simulink model "Simulink_PLC_coder_example"  (R2024a)
settings: Solver=FixedStepDiscrete  StartTime=0.0  StopTime=10  FixedStep=0.0001  RelTol=1e-3
settings Model: Creator=Jan Størbu  LastModifiedBy=Are-Laptop
settings SolverCC: AlgebraicLoopSolver=TrustRegion
settings DataIOCC: ReturnWorkspaceOutputs=off
settings DebuggingCC: UnconnectedInputMsg=warning  UnconnectedOutputMsg=warning  UnconnectedLineMsg=warning  BusObjectLabelMismatch=error  ArithmeticOperatorsInVariantConditions=warning
settings ModelReferenceCC: EnableRefExpFcnMdlSchedulingChecks=on
settings SFSimCC: SimUseLocalCustomCode=off  CustomCodeUndefinedFunction=UseInterfaceOnly
settings RTWCC: RTWUseLocalCustomCode=off  GPUComputeCapability=3.5  DLArmComputeVersion=19.05
settings ConfigComp: PLC_TargetIDE=plcopen  PLC_MultiTBSigbuilderTimeRange=off  PLC_ReuseMLFcnVariable=on  PLC_FoldFBCallOutputVar=off  PLC_RemoveUnusedSSMethodCallArguments=off  PLC_UseCallOutputArgSyntax=off  PLC_EnableUnsignedAndDoubleTypes=off  PLC_EnableUDTSplitting=off  PLC_MaxFieldsInUDT=500  PLC_InlineEnumCastFunction=off  PLC_GenerateReport=off  PLC_LaunchReport=off

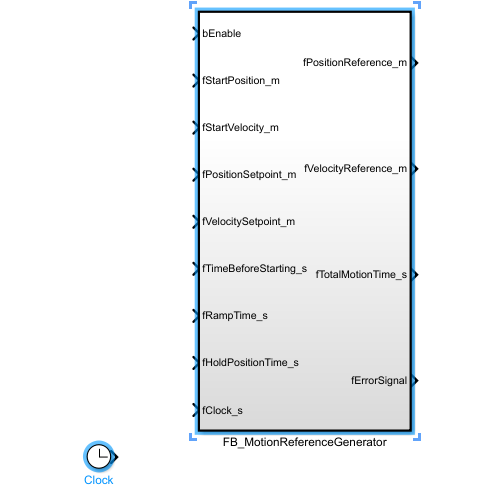
[thumbnail: Simulink's stored preview of the top-level diagram]
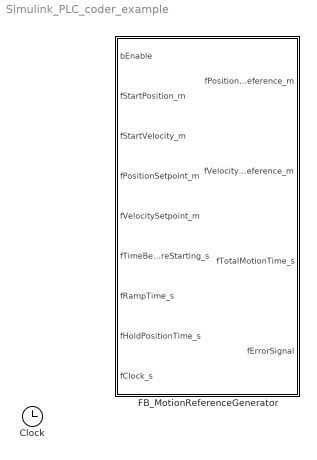
== system Simulink_PLC_coder_example ==
  Clock : Clock
  FB_MotionReferenceGenerator : Subsystem  TreatAsAtomicUnit=on  VariantControl=Ramp_Profile

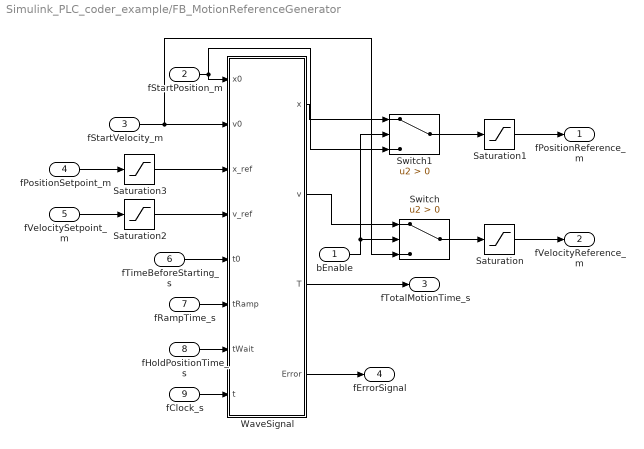
== system Simulink_PLC_coder_example/FB_MotionReferenceGenerator ==
  bEnable : Inport  OutDataTypeStr=boolean
  fStartPosition_m : Inport  Port=2
  fStartVelocity_m : Inport  Port=3
  fPositionSetpoint_m : Inport  Port=4
  fVelocitySetpoint_m : Inport  Port=5
  fTimeBeforeStarting_s : Inport  Port=6
  fRampTime_s : Inport  Port=7
  fHoldPositionTime_s : Inport  Port=8
  fClock_s : Inport  Port=9
  Saturation : Saturate  UpperLimit=0.05  LowerLimit=-0.05
  Saturation1 : Saturate  UpperLimit=0.45  LowerLimit=0
  Saturation2 : Saturate  UpperLimit=0.05  LowerLimit=0
  Saturation3 : Saturate  UpperLimit=0.45  LowerLimit=0
  Switch : Switch  Criteria=u2 > Threshold  SaturateOnIntegerOverflow=off  InputSameDT=off
  Switch1 : Switch  Criteria=u2 > Threshold  SaturateOnIntegerOverflow=off  InputSameDT=off
  WaveSignal : MATLAB Function  TreatAsAtomicUnit=on
  fPositionReference_m : Outport  VectorParamsAs1DForOutWhenUnconnected=off
  fVelocityReference_m : Outport  Port=2  VectorParamsAs1DForOutWhenUnconnected=off
  fTotalMotionTime_s : Outport  Port=3  VectorParamsAs1DForOutWhenUnconnected=off
  fErrorSignal : Outport  Port=4  VectorParamsAs1DForOutWhenUnconnected=off
  wires:
  fClock_s/1 -> WaveSignal/8(t)
  WaveSignal/2(v) -> Switch/1
  Switch/1 -> Saturation/1
  fStartVelocity_m/1 -> Switch/3, WaveSignal/2(v0)
  fTimeBeforeStarting_s/1 -> WaveSignal/5(t0)
  fPositionSetpoint_m/1 -> Saturation3/1
  fHoldPositionTime_s/1 -> WaveSignal/7(tWait)
  fVelocitySetpoint_m/1 -> Saturation2/1
  WaveSignal/1(x) -> Switch1/1
  WaveSignal/3(T) -> fTotalMotionTime_s/1
  fStartPosition_m/1 -> Switch1/3, WaveSignal/1(x0)
  Switch1/1 -> Saturation1/1
  Saturation/1 -> fVelocityReference_m/1
  Saturation2/1 -> WaveSignal/4(v_ref)
  Saturation3/1 -> WaveSignal/3(x_ref)
  fRampTime_s/1 -> WaveSignal/6(tRamp)
  WaveSignal/4(Error) -> fErrorSignal/1
  Saturation1/1 -> fPositionReference_m/1
  bEnable/1 -> Switch1/2, Switch/2

== matlab function Simulink_PLC_coder_example/FB_MotionReferenceGenerator/WaveSignal ==
  data: x0 input; v0 input; x_ref input; x output; v_ref input; t0 input; tRamp input; tWait input; v output; t input; T output; Error output double
function [x,v,T, Error] = fcn(x0,v0, x_ref,v_ref,t0,tRamp,tWait,t)
x_SP = x_ref - x0;
vs=v_ref;
slopeExt=v0-vs;
slopeRetr=-vs-v0;

as = vs/tRamp;
s_acc=(vs^2-v0^2)/as;

tHold=(x_SP-s_acc)/vs;

if tHold < 0 
Error = 1;
else 
Error = 0;
end

t1=tRamp;
t2=tHold; 
t3=tRamp;
t4=tWait;
t5=t1;
t6=t2;
t7=t3;

x = x0;
x1 = x0 + v0*((t0+t1)-t0)-(slopeExt/t1)*((t0+t1)-t0)^2/2;
x2 = x1 + vs*((t0+t1+t2)-(t0+t1)); 
x4 = x_ref - v0*((t0+t1+t2+t3+t4+t5)-(t0+t1+t2+t3+t4))+(slopeRetr/t5)*((t0+t1+t2+t3+t4+t5)-(t0+t1+t2+t3+t4))^2/2; 
x5 = x4-vs*((t0+t1+t2+t3+t4+t5+t6)-(t0+t1+t2+t3+t4+t5));  

if Error == 1
x = x0;
v = v0; 
elseif t>=0 && t<t0
x = x0; 
v = v0;
elseif t>=t0 && t<(t0+t1)
x = x0 + v0*(t-t0)-(slopeExt/t1)*(t-t0)^2/2;
v = v0-(slopeExt/t1)*(t-t0);  
elseif t>=(t0+t1) && t<(t0+t1+t2)
x = x1 + vs*(t-(t0+t1)); 
v = vs; 
elseif t>=(t0+t1+t2) && t<(t0+t1+t2+t3)
x = x2+vs*(t-(t0+t1+t2))+(slopeExt/t3)*(t-(t0+t1+t2))^2/2; 
v = vs+(slopeExt/t3)*(t-(t0+t1+t2));   
elseif t>=(t0+t1+t2+t3) && t<(t0+t1+t2+t3+t4)
x = x_ref;
v = v0;  
elseif t>=(t0+t1+t2+t3+t4) && t<(t0+t1+t2+t3+t4+t5)
x = x_ref - v0*(t-(t0+t1+t2+t3+t4))+(slopeRetr/t5)*(t-(t0+t1+t2+t3+t4))^2/2; 
v = v0+(slopeRetr/t5)*(t-(t0+t1+t2+t3+t4));     
elseif t>=(t0+t1+t2+t3+t4+t5) && t<(t0+t1+t2+t3+t4+t5+t6)
x = x4-vs*(t-(t0+t1+t2+t3+t4+t5));   
v = -vs;    
elseif t>=(t0+t1+t2+t3+t4+t5+t6) && t<(t0+t1+t2+t3+t4+t5+t6+t7)
x = x5-vs*(t-(t0+t1+t2+t3+t4+t5+t6))-(slopeRetr/t3)*(t-(t0+t1+t2+t3+t4+t5+t6))^2/2;    
v = -vs-(slopeRetr/t3)*(t-(t0+t1+t2+t3+t4+t5+t6));     
else 
x = x0;
v = v0; 
end

T = t0+t1+t2+t3+t4+t5+t6+t7;
